simulink model "modellin"  (Simulink 6.0)
settings: Solver=ode45  StartTime=0.0  StopTime=10.0  RelTol=1e-3
settings Model: LastModifiedBy=suraj

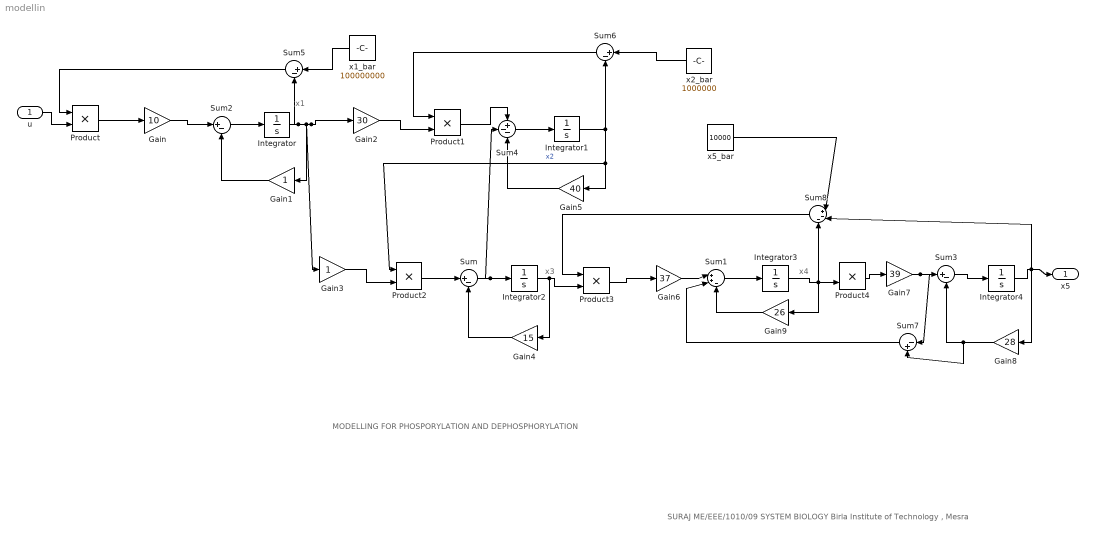
== system modellin ==
  note: x1
  note: x3
  note: x4
  note: MODELLING FOR PHOSPORYLATION AND DEPHOSPHORYLATION
  note: SURAJ
      | ME/EEE/1010/09
      | SYSTEM BIOLOGY
      | Birla Institute of Technology , Mesra
  u : Inport  Port=1  LatchInput=off
  Gain : Gain  Gain=10
  Gain1 : Gain  Orientation=left
  Gain2 : Gain  Gain=30
  Gain3 : Gain
  Gain4 : Gain  Orientation=left  Gain=15
  Gain5 : Gain  Orientation=left  Gain=40
  Gain6 : Gain  Gain=37
  Gain7 : Gain  Gain=39
  Gain8 : Gain  Orientation=left  Gain=28
  Gain9 : Gain  Orientation=left  Gain=26
  Integrator{,1..4} (5 alike) : Integrator
  Product{,1..4} (5 alike) : Product  RndMeth=Zero
  Sum : Sum  Inputs=|+-
  Sum1 : Sum  Inputs=|++-
  Sum2 : Sum  Inputs=|+-
  Sum3 : Sum  Inputs=|+-
  Sum4 : Sum  Inputs=+--
  Sum5 : Sum  Orientation=left  Inputs=|+-
  Sum6 : Sum  Orientation=left  Inputs=|+-
  Sum7 : Sum  Orientation=left  Inputs=|-+
  Sum8 : Sum  Orientation=left  Inputs=|+--
  x1_bar : Constant  Orientation=left  Value=100000000
  x2_bar : Constant  Orientation=left  Value=1000000
  x5_bar : Constant  Value=10000
  x5 : Outport
  wires:
  Product/1 -> Gain/1
  Gain/1 -> Sum2/1
  Sum2/1 -> Integrator/1
  Gain1/1 -> Sum2/2
  Integrator/1 -> Gain1/1, Gain2/1, Gain3/1, Sum5/2
  Gain2/1 -> Product1/2
  Product1/1 -> Sum4/1
  Sum4/1 -> Integrator1/1
  Integrator1/1 -> Gain5/1, Product2/1, Sum6/2  "x2"
  Gain5/1 -> Sum4/3
  Gain3/1 -> Product2/2
  Product2/1 -> Sum/1
  Sum/1 -> Integrator2/1, Sum4/2
  Gain4/1 -> Sum/2
  Integrator2/1 -> Product3/2, Gain4/1
  Product3/1 -> Gain6/1
  Gain6/1 -> Sum1/1
  Integrator4/1 -> x5/1, Gain8/1, Sum8/2
  Sum3/1 -> Integrator4/1
  Gain8/1 -> Sum3/2, Sum7/2
  Gain7/1 -> Sum3/1, Sum7/1
  Product4/1 -> Gain7/1
  Integrator3/1 -> Product4/2, Gain9/1, Sum8/3
  Sum7/1 -> Sum1/2
  Sum1/1 -> Integrator3/1
  u/1 -> Product/2
  Sum5/1 -> Product/1
  Sum6/1 -> Product1/1
  Sum8/1 -> Product3/1
  Gain9/1 -> Sum1/3
  x1_bar/1 -> Sum5/1
  x2_bar/1 -> Sum6/1
  x5_bar/1 -> Sum8/1
